simulink model "segway_TP4_sensors"  (R2016a)
settings: Solver=VariableStepAuto  StartTime=0  StopTime=200  FixedStep=h  RelTol=1e-3
values from neighbouring files (symbols this model uses):
  h = (tf-t0)/N    [init.m]    (also in init_tp3.m)
  L = H/2    (= 0.072)    [matrices_init_tp4_partie3_4.m]
  l = 10    [init.m]    (also in init_TP1.m = 1; init_TP2_controle.m; init_tp3.m = 5)
undefined symbols (not defined in the file or in its folder): DiscIntNeverNeededParam
libraries: simulink x1
settings Model: Creator=fgaribal  LastModifiedBy=fgaribal

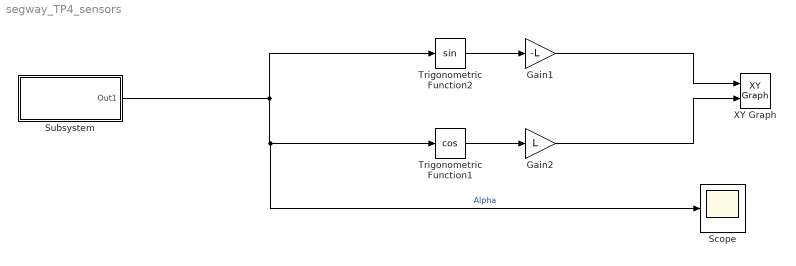
== system segway_TP4_sensors ==
  Gain1 : Gain  Gain=-L
  Gain2 : Gain  Gain=L
  Scope : Scope
  Subsystem : Subsystem
  Trigonometric Function1 : Trigonometry  Operator=cos
  Trigonometric Function2 : Trigonometry
  XY Graph : simulink/Sinks/XY Graph  xmin=-l  xmax=l  ymin=-l  ymax=l  st=-1
  wires:
  Trigonometric Function1/1 -> Gain2/1
  Trigonometric Function2/1 -> Gain1/1
  Gain2/1 -> XY Graph/2
  Gain1/1 -> XY Graph/1
  Subsystem/1(Out1) -> Scope/1, Trigonometric Function1/1, Trigonometric Function2/1  "Alpha"

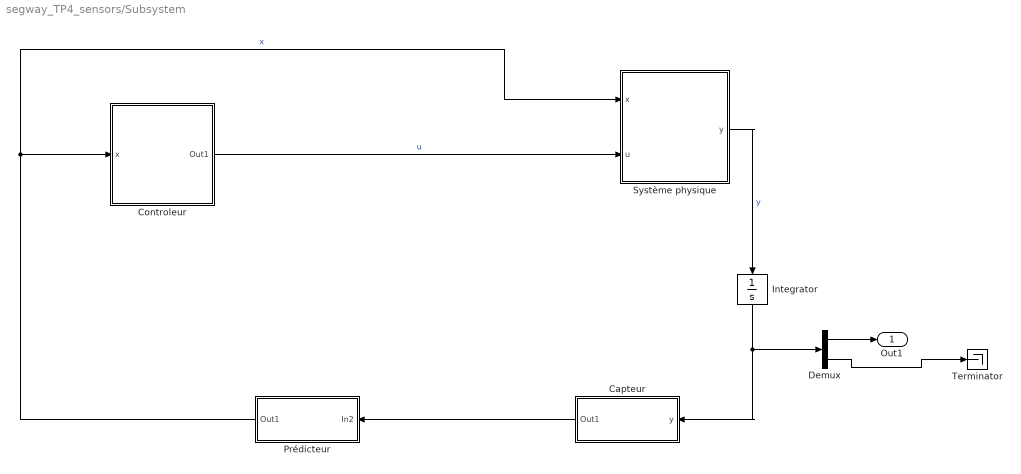
== system segway_TP4_sensors/Subsystem ==
  "Capteur " : Subsystem
  Controleur : Subsystem
  Demux : Demux  Outputs=2
  Integrator : Integrator  InitialCondition=pi/4
  Prédicteur : Subsystem
  Système physique : Subsystem
  Terminator : Terminator
  Out1 : Outport
  wires:
  Controleur/1(Out1) -> Système physique/2(u)  "u"
  Prédicteur/1(Out1) -> Système physique/1(x), Controleur/1(x)  "x"
  Système physique/1(y) -> Integrator/1  "y"
  "Capteur "/1(Out1) -> Prédicteur/1(In2)
  Integrator/1 -> Demux/1, "Capteur "/1(y)
  Demux/1 -> Out1/1
  Demux/2 -> Terminator/1

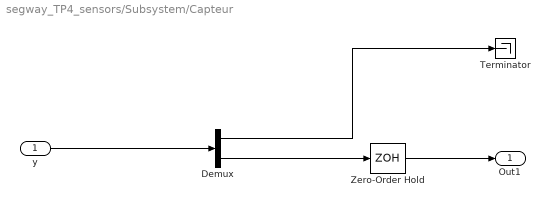
== system segway_TP4_sensors/Subsystem/Capteur  ==
  y : Inport
  Demux : Demux  Outputs=2
  Terminator : Terminator
  Zero-Order Hold : ZeroOrderHold  SampleTime=25*h
  Out1 : Outport
  wires:
  Demux/2 -> Zero-Order Hold/1
  Demux/1 -> Terminator/1
  y/1 -> Demux/1
  Zero-Order Hold/1 -> Out1/1

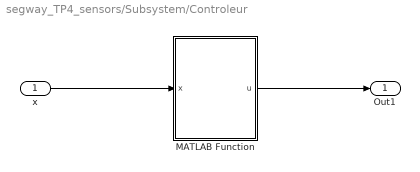
== system segway_TP4_sensors/Subsystem/Controleur ==
  x : Inport
  MATLAB Function : MATLAB Function  TreatAsAtomicUnit=on
  Out1 : Outport
  wires:
  MATLAB Function/1(u) -> Out1/1
  x/1 -> MATLAB Function/1(x)

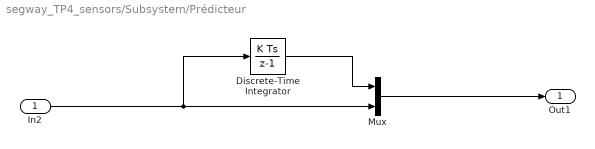
== system segway_TP4_sensors/Subsystem/Prédicteur ==
  In2 : Inport
  Discrete-Time Integrator : DiscreteIntegrator  InitialConditionSetting=State (most efficient)  SampleTime=25*h  ICPrevOutput=DiscIntNeverNeededParam  ICPrevScaledInput=DiscIntNeverNeededParam
  Mux : Mux  Inputs=2
  Out1 : Outport
  wires:
  In2/1 -> Discrete-Time Integrator/1, Mux/2
  Discrete-Time Integrator/1 -> Mux/1
  Mux/1 -> Out1/1

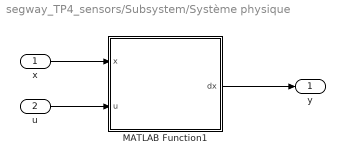
== system segway_TP4_sensors/Subsystem/Système physique ==
  x : Inport
  u : Inport  Port=2
  MATLAB Function1 : MATLAB Function  TreatAsAtomicUnit=on
  y : Outport
  wires:
  MATLAB Function1/1(dx) -> y/1
  x/1 -> MATLAB Function1/1(x)
  u/1 -> MATLAB Function1/2(u)

== matlab function segway_TP4_sensors/Subsystem/Système physique/MATLAB Function1 ==
  data: x input; u input; dx output
%function y = pendule_inverse(x,u)
%    g = 9.81;
%    l = 10;
%    
%    y = zeros(2,1);
%    y(1) = x(2);
%    y(2) = g/l*sin(x(1))-((u*cos(x(1)))/l);
%end


function dx   = fonction( x, u)
%   Dynamic equations of motion of the segway on an axis.
%   Inputs: - x = [theta psi dtheta dpsi]
%               theta: average angle of the wheels      [rad]
%               psi: body pitch angle                   [rad]
%               dtheta: average velocity of the wheels  [rad/s]
%               dpsi: body pitch velocity               [rad/s]
%          - u: DC motor voltage (same value for both motors) [V]

    % State
    psi = x(2);
    dtheta = x(3);
    dpsi = x(4);

    % Parameters
    
    g = 9.81;           % gravity acceleration [m/sec^2]
    m = 0.03;           % wheel weight [kg]
    R = 0.04;           % wheel radius [m]
    Jw = m*R^2/2;       % wheel inertia moment [kg*m^2]
    M = 0.6;            % body weight [kg]
    H = 0.144;          % body height [m]
    L = H/2;            % distance of the center of mass from the wheel axle [m]
    Jpsi = M*L^2/3;     % body pitch inertia [kgm^2]
    Jm = 1e-5;          % DC motor inertia moment [kgm^2]
    Rm = 6.69;          % DC motor resistance [Ohm]
    Kb = 0.468;         % DC motor back EMF constant [Vsec/rad]
    Kt = 0.317;         % DC motor torque constant [Nm/A]
    n = 1;              % gear ratio
    fm = 0.0022;        % friction coefficient between body and DC motor
    fw = 0;             % friction coefficient between wheel and floor
    
    % Equations of motion
    c1 = (2*m+M)*R^2 + 2*Jw + 2*n^2*Jm;
    c2 = M*L*R*cos(psi) - 2*n^2*Jm;
    c3 = -M*L*R*dpsi^2*sin(psi);
    c4 = M*L^2 + Jpsi + 2*n^2*Jm;
    c5 = -M*g*L*sin(psi);

    alpha = Kt/Rm;
    beta = Kt*Kb/Rm + fm;

    Ftheta = alpha*(2*u) - 2*(beta+fw)*dtheta + 2*beta*dpsi;
    Fpsi = -alpha*(2*u) + 2*beta*dtheta - 2*beta*dpsi;

    ddtheta = (c4*c3 - c2*c5 + c4*Ftheta - c2*Fpsi)/(c4*c1 - c2^2);
    ddpsi = (Fpsi- c2*ddtheta - c5)/c4;
    dx = [dtheta dpsi ddtheta ddpsi]';

end

% Matrices of the linearized system
% E = [(2*m+M)*R^2+2*Jw+2*Jm   M*L*R-2*Jm; M*L*R-2*Jm   M*L^2+Jpsi+2*Jm];
% detE = det(E);

% alpha = Kt/Rm;
% beta = Kt*Kb/Rm + fm;

% A32 = -M*g*L*E(1,2)/detE;
% A42 = M*g*L*E(1,1)/detE;
% A33 = -(beta*E(2,2)+2*beta*E(1,2))/detE;
% A43 = (beta*E(1,2)+2*beta*E(1,1))/detE;
% A34 = beta*(E(2,2)+2*E(1,2))/detE;
% A44 = -beta*(E(1,2)+2*E(1,1))/detE;

% B3 = alpha*(E(2,2)/2+E(1,2))/detE;
% B4 = -alpha*(E(1,2)/2+E(1,1))/detE;

% A = [0 0 1 0;0 0 0 1; 0 A32 A33 A34; 0 A42 A43 A44];
% B = [0 0 2*B3 2*B4];

== matlab function segway_TP4_sensors/Subsystem/Controleur/MATLAB Function ==
  data: x input; u output
function u = calcul_u(x)
    ue = 0;
    xe = [0;0];
    K = [20;10];
    
    u = ue + K'*(x-xe);
end
